simulink model "Simulink_ControllerARMAX"  (R2020b)
settings: Solver=VariableStepAuto  StartTime=0.0  StopTime=2000  RelTol=1e-3
values from neighbouring files (symbols this model uses):
  c0_Gc = (S0 + S1 + S2)/(1+r0)    [Controller_ARMAX_BlaneRev.m]    (also in Controller_SS_BlaneRev.m)
  c0_Gff = (T_S2 + T_S1 + T_S0)/(1+r0)    [Controller_ARMAX_BlaneRev.m]    (also in Controller_SS_BlaneRev.m)
  Gp = tf(sysARMAX)    [Controller_ARMAX_BlaneRev.m]    (also in Controller_SS_BlaneRev.m = tf(B, A, Ts2); Controller_TF_BlaneRev.m = tf(sysTF))
  K_ant = 10    [Controller_ARMAX_BlaneRev.m]
  PD_den = [1, r0]    [Controller_ARMAX_BlaneRev.m]    (also in Controller_SS_BlaneRev.m)
  PD_SR_num = [d1_Gc, d0_Gc]    [Controller_ARMAX_BlaneRev.m]    (also in Controller_SS_BlaneRev.m)
  PD_TR_num = [d1_Gff, d0_Gff]    [Controller_ARMAX_BlaneRev.m]    (also in Controller_SS_BlaneRev.m)
  R = [1, r0-1, r0]    [Controller_ARMAX_BlaneRev.m]    (also in Controller_SS_BlaneRev.m = [1, r0-1, -r0]; Controller_TF_BlaneRev.m = [1, -1])
  S = [S2, S1, S0]    [Controller_ARMAX_BlaneRev.m]    (also in Controller_SS_BlaneRev.m; Controller_TF_BlaneRev.m = [S1, S0])
  T = t_o*A_o    [Controller_ARMAX_BlaneRev.m]    (also in Controller_SS_BlaneRev.m; Controller_TF_BlaneRev.m; systemIdentification_BlaneRev.m = flip(T))
  Ts = .4    (= 0.4)    [Controller_ARMAX_BlaneRev.m]    (also in Controller_SS_BlaneRev.m; Controller_TF_BlaneRev.m; systemIdentification_47414_Blane.m = 0.2; systemIdentification_48404_Blane.m = 1)
undefined symbols (not defined in the file or in its folder): DiscIntNeverNeededParam
settings Model: Creator=Blane Brinkley  LastModifiedBy=Blane Brinkley

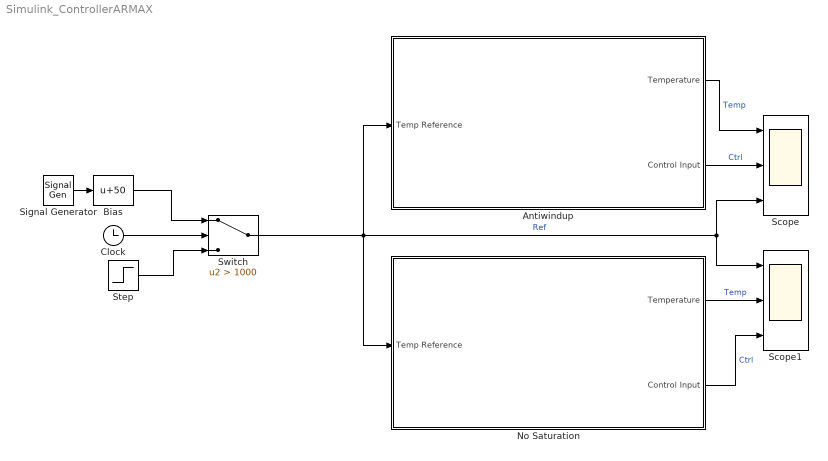
== system Simulink_ControllerARMAX ==
  Antiwindup : Subsystem
  Bias : Bias  Bias=50
  Clock : Clock
  No Saturation : Subsystem
  Scope : Scope  NumInputPorts=3
  Scope1 : Scope  NumInputPorts=3
  Signal Generator : SignalGenerator  WaveForm=square  Amplitude=10  Frequency=1/1800
  Step : Step  Time=500  After=50  SampleTime=Ts
  Switch : Switch  Criteria=u2 > Threshold  Threshold=1000
  wires:
  Signal Generator/1 -> Bias/1
  Antiwindup/1("Temperature ") -> Scope/1  "Temp"
  Antiwindup/2("Control Input ") -> Scope/2  "Ctrl"
  Step/1 -> Switch/3
  Switch/1 -> No Saturation/1(Temp Reference), Scope1/1, Scope/3, Antiwindup/1(Temp Reference)  "Ref"
  Bias/1 -> Switch/1
  Clock/1 -> Switch/2
  No Saturation/1("Temperature ") -> Scope1/2  "Temp"
  No Saturation/2("Control Input ") -> Scope1/3  "Ctrl"

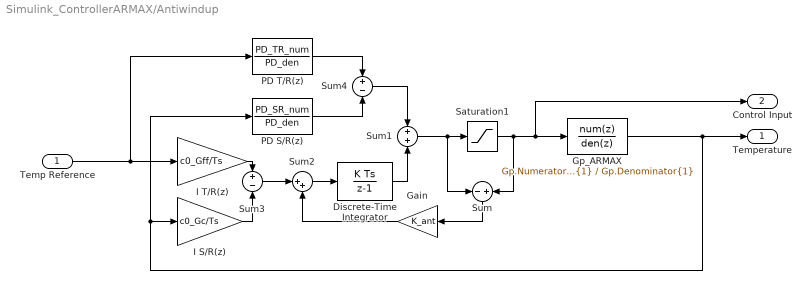
== system Simulink_ControllerARMAX/Antiwindup ==
  Temp Reference : Inport
  Discrete-Time Integrator : DiscreteIntegrator  SampleTime=Ts  ICPrevOutput=DiscIntNeverNeededParam  ICPrevScaledInput=DiscIntNeverNeededParam
  Gain : Gain  Gain=K_ant
  Gp_ARMAX : DiscreteTransferFcn  Numerator=Gp.Numerator{1}  Denominator=Gp.Denominator{1}  SampleTime=Ts
  I S/R(z) : Gain  Gain=c0_Gc/Ts
  I T/R(z) : Gain  Gain=c0_Gff/Ts
  PD S/R(z) : DiscreteTransferFcn  Numerator=PD_SR_num  Denominator=PD_den
  PD T/R(z) : DiscreteTransferFcn  Numerator=PD_TR_num  Denominator=PD_den
  Saturation1 : Saturate  UpperLimit=100  LowerLimit=0
  Sum : Sum  Inputs=-+
  Sum1 : Sum
  Sum2 : Sum  Inputs=|++
  Sum3 : Sum  Inputs=+-
  Sum4 : Sum  Inputs=+-
  "Temperature " : Outport
  "Control Input " : Outport  Port=2
  wires:
  Sum3/1 -> Sum2/1
  I S/R(z)/1 -> Sum3/2
  Sum2/1 -> Discrete-Time Integrator/1
  Gp_ARMAX/1 -> I S/R(z)/1, PD S/R(z)/1, "Temperature "/1
  I T/R(z)/1 -> Sum3/1
  Discrete-Time Integrator/1 -> Sum1/2
  Sum1/1 -> Sum/1, Saturation1/1
  Sum/1 -> Gain/1
  Sum4/1 -> Sum1/1
  PD S/R(z)/1 -> Sum4/2
  Saturation1/1 -> "Control Input "/1, Gp_ARMAX/1, Sum/2
  PD T/R(z)/1 -> Sum4/1
  Gain/1 -> Sum2/2
  Temp Reference/1 -> PD T/R(z)/1, I T/R(z)/1

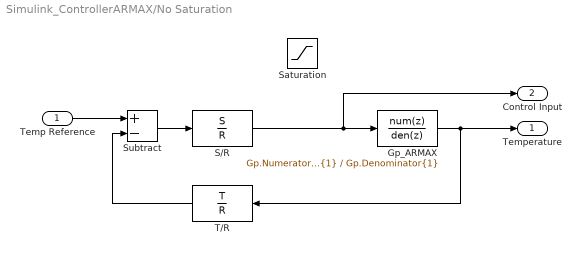
== system Simulink_ControllerARMAX/No Saturation ==
  Temp Reference : Inport
  Gp_ARMAX : DiscreteTransferFcn  Numerator=Gp.Numerator{1}  Denominator=Gp.Denominator{1}  SampleTime=Ts
  S/R : DiscreteTransferFcn  Numerator=S  Denominator=R
  Saturation : Saturate  UpperLimit=100  LowerLimit=0
  Subtract : Sum  Inputs=+-
  T/R : DiscreteTransferFcn  Numerator=T  Denominator=R
  "Temperature " : Outport
  "Control Input " : Outport  Port=2
  wires:
  Gp_ARMAX/1 -> "Temperature "/1, T/R/1
  Temp Reference/1 -> Subtract/1
  S/R/1 -> "Control Input "/1, Gp_ARMAX/1
  Subtract/1 -> S/R/1
  T/R/1 -> Subtract/2
